simulink model "clap_on_off_arduino_uno_R2022a_Linux"  (R2022a)
settings: Solver=FixedStepDiscrete  StartTime=0.0  StopTime=inf  FixedStep=0.005  RelTol=1e-3  EnableMultiTasking=on
libraries: arduinolib x4, simulink_extras x1, eeGeneralControl x1
settings Model: ExtModeTrigDuration=2  Creator=john  LastModifiedBy=byoun
settings SolverCC: AutoInsertRateTranBlk=on
settings OptimizationCC: EnhancedBackFolding=on  PassReuseOutputArgsAs=Individual arguments  ZeroExternalMemoryAtStartup=off  ZeroInternalMemoryAtStartup=off  MaxStackSize=64  OptimizeBlockOrder=speed  DifferentSizesBufferReuse=on  OptimizationCustomize=off  EfficientTunableParamExpr=on
settings DebuggingCC: ParameterTunabilityLossMsg=error  UnconnectedInputMsg=warning  UnconnectedOutputMsg=warning  UnconnectedLineMsg=warning
settings HardwareCC: ProdBitPerInt=16  ProdBitPerPointer=16  ProdBitPerSizeT=16  ProdBitPerPtrDiffT=16  ProdLargestAtomicFloat=None  ProdWordSize=8  ProdHWDeviceType=Atmel->AVR
settings SFSimCC: MATLABDynamicMemAlloc=off
settings RTWCC: SystemTargetFile=ert.tlc  HardwareBoard=Arduino Uno  TemplateMakefile=ert_default_tmf  Toolchain=Arduino AVR  BuildConfiguration=Faster Runs  DLArmComputeVersion=19.05
settings CodeAppCC: ForceParamTrailComments=on  IgnoreCustomStorageClasses=off  OperatorAnnotations=on  SimulinkDataObjDesc=on  SFDataObjDesc=on  InsertBlockDesc=on
settings ERTTargetCC: SupportContinuousTime=on  SupportVariableSizeSignals=on  ExtModeTransport=3  ExtModeStaticAlloc=on  ExtModeStaticAllocSize=250  ExtModeMexFile=ext_xcp  ExtModeIntrfLevel=Level2 - Open

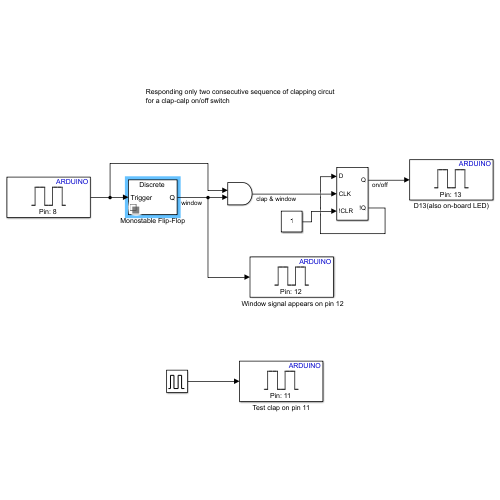
[thumbnail: Simulink's stored preview of the top-level diagram]
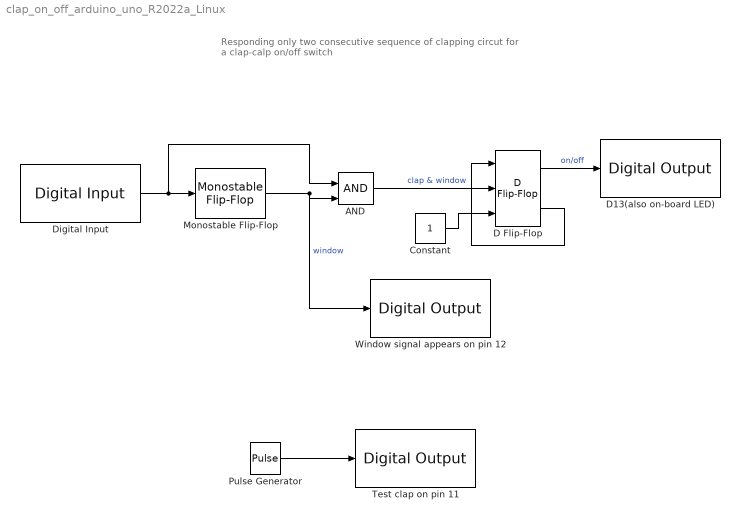
== system clap_on_off_arduino_uno_R2022a_Linux ==
  note: Responding only two consecutive sequence of clapping circut
      | for a clap-calp on/off switch
  " Window signal appears on pin 12" : arduinolib/Digital Output  pinNumber=12  Direction=output  blockPlatform=arduino
  AND : Logic  IconShape=distinctive  AllPortsSameDT=off  OutDataTypeStr=boolean
  Constant : Constant
  D Flip-Flop : simulink_extras/Flip Flops/D Flip-Flop
  D13(also on-board LED) : arduinolib/Digital Output  pinNumber=13  Direction=output  blockPlatform=arduino
  Digital Input : arduinolib/Digital Input  pinNumber=8  mode=Default  Direction=input  SampleTime=0.005  blockPlatform=arduino
  Monostable Flip-Flop : eeGeneralControl/Monostable Flip-Flop  VariantControl=Variant1  LabelModeActiveChoice=Discrete  ChangeType=Falling edge  x0=0  Td=0.08  Ts=0.005
      settings: SourceProductBaseCode=PS
  Pulse Generator : DiscretePulseGenerator  PulseType=Time based  Period=0.05  PulseWidth=10
  Test clap on pin 11 : arduinolib/Digital Output  pinNumber=11  Direction=output  blockPlatform=arduino
  wires:
  D Flip-Flop/2 -> D Flip-Flop/1
  Constant/1 -> D Flip-Flop/3
  AND/1 -> D Flip-Flop/2  "clap & window"
  Monostable Flip-Flop/1 -> AND/2, " Window signal appears on pin 12"/1  "window"
  D Flip-Flop/1 -> D13(also on-board LED)/1  "on/off"
  Digital Input/1 -> Monostable Flip-Flop/1, AND/1
  Pulse Generator/1 -> Test clap on pin 11/1
